simulink subsystem "EvitaParedes"  (R2023b)
settings: Solver=VariableStepAuto  StartTime=0.0  StopTime=10.0  RelTol=1e-3
settings Model: Creator=pablo  LastModifiedBy=pablo

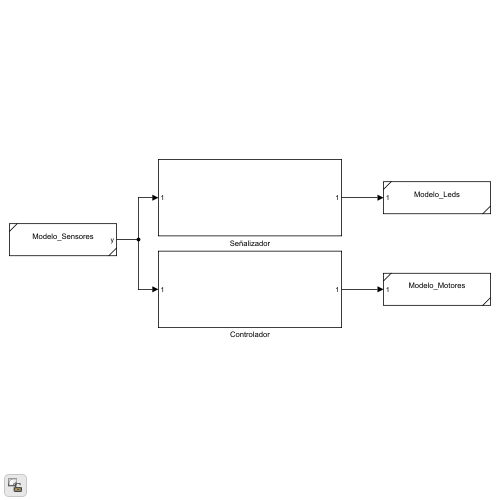
[thumbnail: Simulink's stored preview of the top-level diagram]
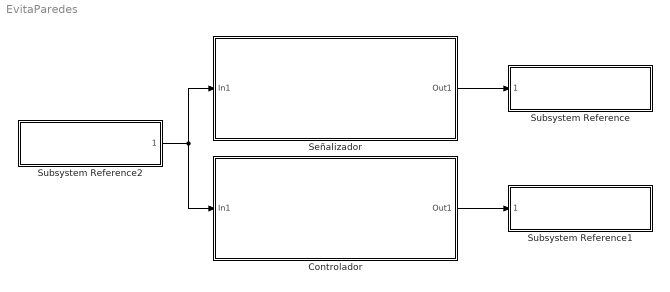
== system EvitaParedes ==
  Controlador : Subsystem
  Señalizador : Subsystem
  Subsystem Reference : Subsystem  ReferencedSubsystem=Modelo_Leds
  Subsystem Reference1 : Subsystem  ReferencedSubsystem=Modelo_Motores
  Subsystem Reference2 : Subsystem  ReferencedSubsystem=Modelo_Sensores
  wires:
  Señalizador/1(Out1) -> Subsystem Reference/1
  Controlador/1(Out1) -> Subsystem Reference1/1
  Subsystem Reference2/1 -> Señalizador/1(In1), Controlador/1(In1)

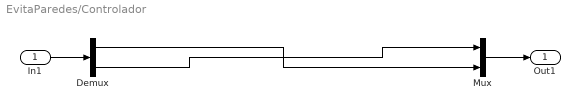
== system EvitaParedes/Controlador ==
  In1 : Inport
  Demux : Demux  Outputs=2
  Mux : Mux  Inputs=2
  Out1 : Outport
  wires:
  Mux/1 -> Out1/1
  In1/1 -> Demux/1
  Demux/1 -> Mux/2
  Demux/2 -> Mux/1

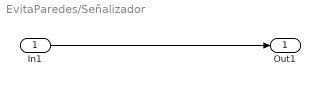
== system EvitaParedes/Señalizador ==
  In1 : Inport
  Out1 : Outport
  wires:
  In1/1 -> Out1/1
